simulink model "RM3_rackAndPinion_w_PEC"  (R2024b)
settings: Solver=ode4  StartTime=0  StopTime=200  FixedStep=0.001  MaxStep=0.001  RelTol=1e-3
values from neighbouring files (symbols this model uses):
  simu = simulationClass()    [wecSimInputFile.m]
undefined symbols (not defined in the file or in its folder): body, constraint, diodeA, diodeB1, diodeB2, diodeC, fsw, geometry, heatSinkCth, heatSinkRth, hydroData, igbtA, igbtB1, igbtB2, igbtC, igbtRth, numParallel, pmsg, pto, Vdc, wec, wi
libraries: WECSim_Lib_Body_Elements x2, WECSim_Lib_Frames x1, WECSim_Lib_Constraints x1, WECSim_Lib_PTOs x1
settings Model: Creator=smbar  LastModifiedBy=smbar
settings SolverCC: ZeroCrossControl=DisableAll  AutoInsertRateTranBlk=on
settings DataIOCC: ReturnWorkspaceOutputs=off
settings OptimizationCC: SimCompilerOptimization=on
settings ExplorerConfigSet: SimMechanicsOpenEditorOnUpdate=off

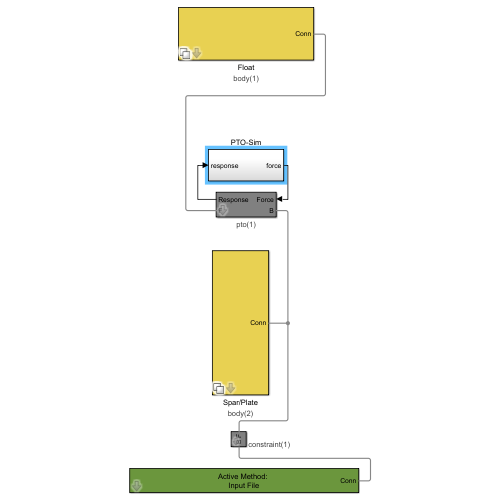
[thumbnail: Simulink's stored preview of the top-level diagram]
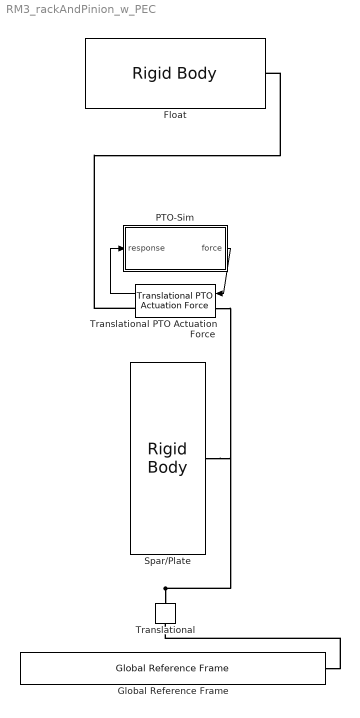
== system RM3_rackAndPinion_w_PEC ==
  Float : WECSim_Lib_Body_Elements/Rigid Body  body=body(1)  h5File=hydroData/*.h5  geometryFile=geometry/*.stl  mass=0  inertia=0 0 0  inertiaProducts=0 0 0  nonHydro=0  nonlinearHydro=0  centerGravity=0 0 0  centerBuoyancy=0 0 0  dof=6  volume=0  QTFs=0  displacement=0 0 0  axis=0 1 0  angle=0  option=0  cd=0 0 0  ca=0 0 0  area=0 0 0  VME=0  rgME=0 0 0  z=0 0 1
  Global Reference Frame : WECSim_Lib_Frames/Global Reference Frame  waves=waves  simu=simu  InputMethod=Input File  InputFile=wecSimInputFile.m  mode=normal  explorer=off  solver=ode4  startTime=0  rampTime=100  endTime=400  dt=0.1  cicEndTime=60  stateSpace=0  WaveClass=regular  height=2.5  period=8  elevationFile=NOT DEFINED  spectrumFile=NOT DEFINED  direction=0  spread=1  spectrumType=NOT DEFINED  phaseSeed=0  option=EqualEnergy
  PTO-Sim : Subsystem
  Spar/Plate : WECSim_Lib_Body_Elements/Rigid Body  body=body(2)  h5File=hydroData/*.h5  geometryFile=geometry/*.stl  mass=0  inertia=0 0 0  inertiaProducts=0 0 0  nonHydro=0  nonlinearHydro=0  centerGravity=0 0 0  centerBuoyancy=0 0 0  dof=6  volume=0  QTFs=0  displacement=0 0 0  axis=0 1 0  angle=0  option=0  cd=0 0 0  ca=0 0 0  area=0 0 0  VME=0  rgME=0 0 0  z=0 0 1
  Translational : WECSim_Lib_Constraints/Translational  constraint=constraint(1)  loc="0  0  0"  displacement=0 0 0  y=0 1 0  z=0 0 1  upperLimitSpecify=off  upperLimitBound=0  upperLimitTransitionRegionWidth=0  upperLimitStiffness=0  upperLimitDamping=0  lowerLimitSpecify=off  lowerLimitBound=0  lowerLimitTransitionRegionWidth=0  lowerLimitStiffness=0  lowerLimitDamping=0
      settings: AttributesFormatString=%<constraint>
  Translational PTO Actuation Force : WECSim_Lib_PTOs/Translational PTO Actuation Force  pto=pto(1)  loc="0  0  0"  stiffness=0  damping=0  equilibriumPosition=0  pretension=0  displacement=0 0 0  y=0 1 0  z=0 0 1  upperLimitSpecify=off  upperLimitBound=0  upperLimitTransitionRegionWidth=0  upperLimitStiffness=0  upperLimitDamping=0  lowerLimitSpecify=off  lowerLimitBound=0  lowerLimitTransitionRegionWidth=0  lowerLimitStiffness=0  lowerLimitDamping=0
      settings: AttributesFormatString=%<pto>
  wires:
  Translational PTO Actuation Force/1 -> PTO-Sim/1(response)
  PTO-Sim/1(force) -> Translational PTO Actuation Force/1
  connections:
  Translational/RConn1 -- Spar/Plate/RConn1 -- Translational PTO Actuation Force/LConn1
  Global Reference Frame/RConn1 -- Translational/LConn1
  Translational PTO Actuation Force/RConn1 -- Float/RConn1

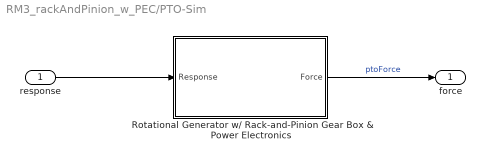
== system RM3_rackAndPinion_w_PEC/PTO-Sim ==
  response : Inport
  Rotational Generator w/ Rack-and-Pinion Gear Box & Power Electronics : Subsystem
  force : Outport  VectorParamsAs1DForOutWhenUnconnected=off
  wires:
  response/1 -> Rotational Generator w/ Rack-and-Pinion Gear Box & Power Electronics/1(Response)
  Rotational Generator w/ Rack-and-Pinion Gear Box & Power Electronics/1(Force) -> force/1  "ptoForce"

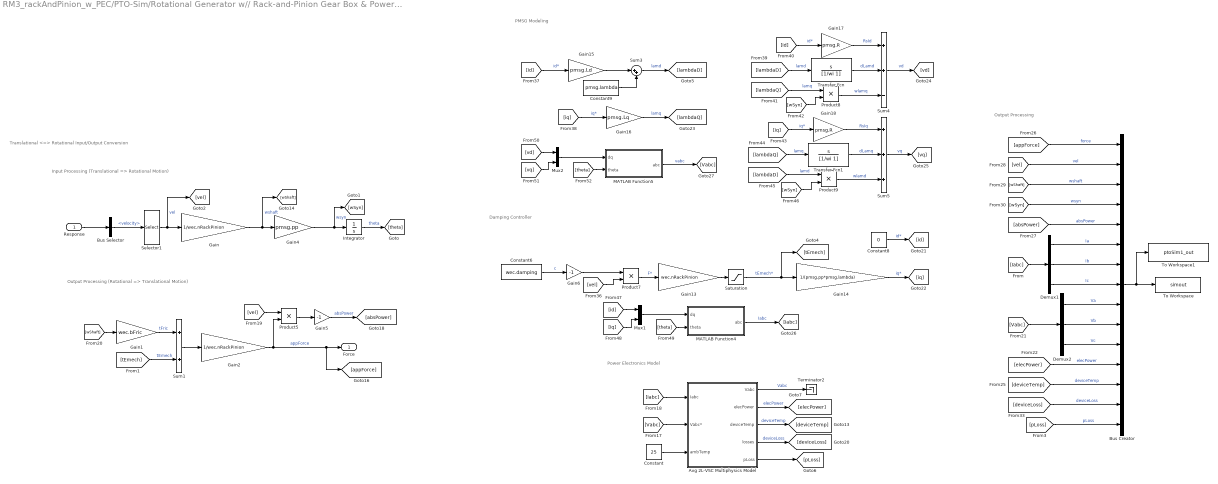
== system RM3_rackAndPinion_w_PEC/PTO-Sim/Rotational Generator w// Rack-and-Pinion Gear Box & Power Electronics ==
  note: Damping Controller
  note: PMSG Modeling
  note: Output Processing
  note: Output Processing (Rotational => Translational Motion)
  note: Input Processing (Translational => Rotational Motion)
  note: Translational <=> Rotational Input/Output Conversion
  note: Power Electronics Model
  Response : Inport
  Avg 2L-VSC Multiphysics Model : Subsystem
  Bus Creator : BusCreator  Inputs=15
  Bus Selector : BusSelector  OutputSignals=velocity
  Constant : Constant  Value=25
  Constant6 : Constant  Value=wec.damping
  Constant8 : Constant  Value=0
  Constant9 : Constant  Value=pmsg.lambda
  Demux1 : Demux  Outputs=3
  Demux2 : Demux  Outputs=3
  Gain : Gain  Gain=1/wec.nRackPinion
  Gain1 : Gain  Gain=wec.bFric
  Gain13 : Gain  Gain=wec.nRackPinion
  Gain14 : Gain  Gain=1/(pmsg.pp*pmsg.lambda)
  Gain15 : Gain  Gain=pmsg.Ld
  Gain16 : Gain  Gain=pmsg.Lq
  Gain17 : Gain  Gain=pmsg.R
  Gain18 : Gain  Gain=pmsg.R
  Gain2 : Gain  Gain=1/wec.nRackPinion
  Gain4 : Gain  Gain=pmsg.pp
  Gain5 : Gain  Gain=-1
  Gain6 : Gain  Gain=-1
  Integrator : Integrator  WrapState=on  WrappedStateUpperValue=2*pi  WrappedStateLowerValue=0
  MATLAB Function4 : MATLAB Function  TreatAsAtomicUnit=on
  MATLAB Function5 : MATLAB Function  TreatAsAtomicUnit=on
  Mux1 : Mux  Inputs=2
  Mux2 : Mux  Inputs=2
  Product{5,7..9} (4 alike) : Product
  Saturation : Saturate  UpperLimit=pmsg.tRated  LowerLimit=-pmsg.tRated
  Selector1 : Selector  InputPortWidth=6  IndexOptions=Index vector (dialog)  Indices=3  OutputSizes=1
  Sum1 : Sum
  Sum3 : Sum  Inputs=|++
  Sum4 : Sum  Inputs=++-
  Sum5 : Sum  Inputs=+++
  Terminator2 : Terminator
  To Workspace : ToWorkspace  VariableName=simout  SaveFormat=Timeseries  SampleTime=-1
  To Workspace1 : ToWorkspace  VariableName=ptoSim1_out  SaveFormat=Structure With Time  SampleTime=simu.dtOut
  Transfer Fcn : TransferFcn  Numerator=[1 0]  Denominator=[1/wi 1]
  Transfer Fcn1 : TransferFcn  Numerator=[1 0]  Denominator=[1/wi 1]
  Force : Outport
  wires:
  Bus Selector/1 -> Selector1/1  "<velocity>"
  Response/1 -> Bus Selector/1
  Selector1/1 -> [vel], Gain/1  "vel"
  Gain4/1 -> Integrator/1, [wSyn]  "wsyn"
  Integrator/1 -> [theta]  "theta"
  [wShaft] -> Gain1/1
  Gain1/1 -> Sum1/1  "tFric"
  Gain2/1 -> [appForce], Force/1, Product5/2  "appForce"
  Sum1/1 -> Gain2/1
  [tEmech] -> Sum1/2  "tEmech"
  [Vabc] -> Avg 2L-VSC Multiphysics Model/2(Vabc*)
  [Iabc] -> Avg 2L-VSC Multiphysics Model/1(Iabc)
  Constant/1 -> Avg 2L-VSC Multiphysics Model/3(ambTemp)
  Avg 2L-VSC Multiphysics Model/1(Vabc) -> Terminator2/1  "Vabc"
  Avg 2L-VSC Multiphysics Model/2(elecPower) -> [elecPower]  "elecPower"
  Avg 2L-VSC Multiphysics Model/3(deviceTemp) -> [deviceTemp]  "deviceTemp"
  Gain/1 -> [wShaft], Gain4/1  "wshaft"
  [vel] -> Product5/1
  Product5/1 -> Gain5/1
  Gain5/1 -> [absPower]  "absPower"
  Bus Creator/1 -> To Workspace1/1, To Workspace/1
  [Iabc] -> Demux1/1
  [Vabc] -> Demux2/1
  Demux2/1 -> Bus Creator/9  "Va"
  [elecPower] -> Bus Creator/12  "elecPower"
  [deviceTemp] -> Bus Creator/13  "deviceTemp"
  Demux2/2 -> Bus Creator/10  "Vb"
  Demux2/3 -> Bus Creator/11  "Vc"
  Demux1/2 -> Bus Creator/7  "Ib"
  Demux1/1 -> Bus Creator/6  "Ia"
  Demux1/3 -> Bus Creator/8  "Ic"
  [appForce] -> Bus Creator/1  "force"
  [vel] -> Bus Creator/2  "vel"
  [wShaft] -> Bus Creator/3  "wshaft"
  [wSyn] -> Bus Creator/4  "wsyn"
  [absPower] -> Bus Creator/5  "absPower"
  [pLoss] -> Bus Creator/15  "pLoss"
  Avg 2L-VSC Multiphysics Model/4(losses) -> [deviceLoss]  "deviceLoss"
  [deviceLoss] -> Bus Creator/14  "deviceLoss"
  [vel] -> Product7/2
  Product7/1 -> Gain13/1  "F*"
  Gain13/1 -> Saturation/1
  Gain14/1 -> [iq]  "iq*"
  [id] -> Gain15/1  "id*"
  Gain15/1 -> Sum3/1
  Constant9/1 -> Sum3/2
  Sum3/1 -> [lambdaD]  "lamd"
  Gain16/1 -> [lambdaQ]  "lamq"
  Constant8/1 -> [id]  "id*"
  [iq] -> Gain16/1  "iq*"
  [lambdaD] -> Transfer Fcn/1  "lamd"
  Transfer Fcn/1 -> Sum4/2  "dLamd"
  [id] -> Gain17/1  "id*"
  [lambdaQ] -> Product8/1  "lamq"
  [wSyn] -> Product8/2
  Gain17/1 -> Sum4/1  "RsId"
  Product8/1 -> Sum4/3  "wlamq"
  Sum4/1 -> [vd]  "vd"
  [iq] -> Gain18/1  "iq*"
  [lambdaQ] -> Transfer Fcn1/1  "lamq"
  Product9/1 -> Sum5/3  "wlamd"
  Transfer Fcn1/1 -> Sum5/2  "dLamq"
  Gain18/1 -> Sum5/1  "RsIq"
  [lambdaD] -> Product9/1  "lamd"
  [wSyn] -> Product9/2
  Sum5/1 -> [vq]  "vq"
  [iq] -> Mux1/2
  [id] -> Mux1/1
  Mux1/1 -> MATLAB Function4/1(dq)
  [theta] -> MATLAB Function4/2(theta)
  MATLAB Function4/1(abc) -> [Iabc]  "Iabc"
  [theta] -> MATLAB Function5/2(theta)
  [vd] -> Mux2/1
  Mux2/1 -> MATLAB Function5/1(dq)
  [vq] -> Mux2/2
  MATLAB Function5/1(abc) -> [Vabc]  "vabc"
  Gain6/1 -> Product7/1
  Constant6/1 -> Gain6/1  "c"
  Saturation/1 -> [tEmech], Gain14/1  "tEmech*"
  Avg 2L-VSC Multiphysics Model/5(pLoss) -> [pLoss]

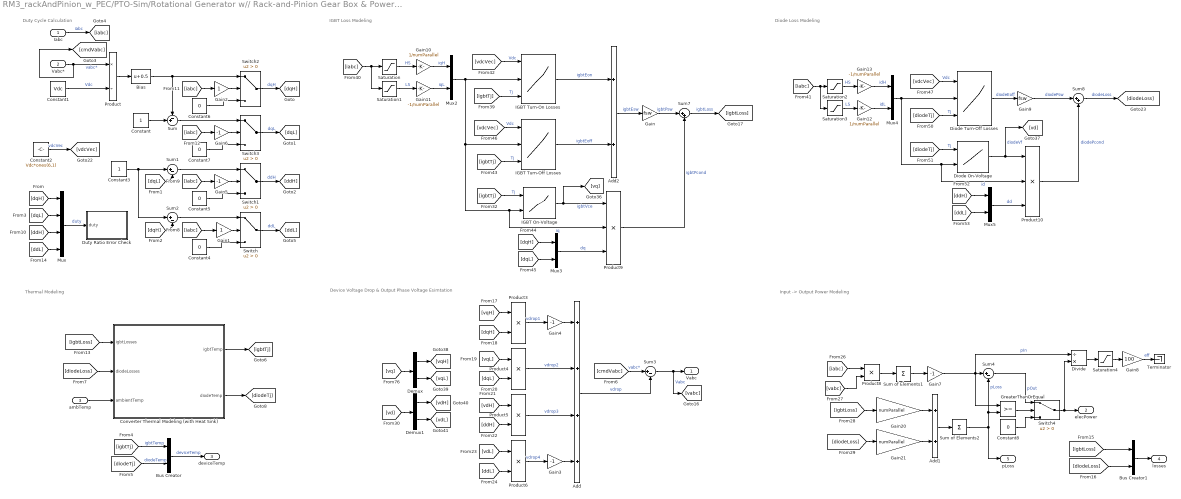
== system RM3_rackAndPinion_w_PEC/PTO-Sim/Rotational Generator w// Rack-and-Pinion Gear Box & Power Electronics/Avg 2L-VSC Multiphysics Model ==
  note: Thermal Modeling
  note: Diode Loss Modeling
  note: IGBT Loss Modeling
  note: Input -> Output Power Modeling
  note: Device Voltage Drop & Output Phase Voltage Esimtation
  note: Duty Cycle Calculation
  Iabc : Inport
  Vabc* : Inport  Port=2
  ambTemp : Inport  Port=3
  Add : Sum  Inputs=++++
  Add1 : Sum
  Add2 : Sum
  Bias : Bias  Bias=0.5  SaturateOnIntegerOverflow=off
  Bus Creator : BusCreator  Inputs=2
  Bus Creator1 : BusCreator  Inputs=2
  Constant : Constant
  Constant1 : Constant  Value=Vdc
  Constant2 : Constant  Value=Vdc*ones(6,1)
  Constant3 : Constant
  Constant{4..8} (5 alike) : Constant  Value=0
  Converter Thermal Modeling (with Heat Sink) : Subsystem
  Demux : Demux  Outputs=2
  Demux1 : Demux  Outputs=2
  Diode On-Voltage : Lookup_n-D  DataSpecification=Lookup table object  LookupTableObject=diodeVonLUT  BreakpointsForDimension3=[5, 7]  Table=reshape(repmat([4 5 6;16 19 20;10 18 23],1,2),[3,3,2])  InternalRulePriority=Speed  RndMeth=Simplest
      settings: InputPortMap=u0,u1
  Diode Turn-Off Losses : Lookup_n-D  NumberOfTableDimensions=3  DataSpecification=Lookup table object  LookupTableObject=diodeEoffLUT  BreakpointsForDimension3=[5, 7]  Table=reshape(repmat([4 5 6;16 19 20;10 18 23],1,2),[3,3,2])  InternalRulePriority=Speed  RndMeth=Simplest
      settings: InputPortMap=u0,u1,u2
  Divide : Product  Inputs=/*
  Duty Ratio Error Check : Subsystem
  Gain : Gain  Gain=fsw
  Gain1 : Gain
  Gain10 : Gain  Gain=1/numParallel
  Gain11 : Gain  Gain=-1/numParallel
  Gain12 : Gain  Gain=1/numParallel
  Gain13 : Gain  Gain=-1/numParallel
  Gain2 : Gain
  Gain20 : Gain  Gain=numParallel
  Gain21 : Gain  Gain=numParallel
  Gain{3..7} (5 alike) : Gain  Gain=-1
  Gain8 : Gain  Gain=100
  Gain9 : Gain  Gain=fsw
  GreaterThanOrEqual : RelationalOperator  OutDataTypeStr=boolean  RndMeth=Simplest  InputSameDT=off
  IGBT On-Voltage : Lookup_n-D  DataSpecification=Lookup table object  LookupTableObject=igbtVonLUT  BreakpointsForDimension3=[5, 7]  Table=reshape(repmat([4 5 6;16 19 20;10 18 23],1,2),[3,3,2])  InternalRulePriority=Speed  RndMeth=Simplest
      settings: InputPortMap=u0,u1
  IGBT Turn-Off Losses : Lookup_n-D  NumberOfTableDimensions=3  DataSpecification=Lookup table object  LookupTableObject=igbtEoffLUT  BreakpointsForDimension3=[5, 7]  Table=reshape(repmat([4 5 6;16 19 20;10 18 23],1,2),[3,3,2])  InternalRulePriority=Speed  RndMeth=Simplest
      settings: InputPortMap=u0,u1,u2
  IGBT Turn-On Losses : Lookup_n-D  NumberOfTableDimensions=3  DataSpecification=Lookup table object  LookupTableObject=igbtEonLUT  BreakpointsForDimension3=[5, 7]  Table=reshape(repmat([4 5 6;16 19 20;10 18 23],1,2),[3,3,2])  InternalRulePriority=Speed  RndMeth=Simplest
      settings: InputPortMap=u0,u1,u2
  Mux : Mux  Inputs=[3 3 3 3]
  Mux{2..5} (4 alike) : Mux  Inputs=2
  Product : Product  Inputs=*/
  Product10 : Product  Inputs=3
  Product{3..6,8} (5 alike) : Product
  Product9 : Product  Inputs=3
  Saturation : Saturate  UpperLimit=inf  LowerLimit=0
  Saturation1 : Saturate  UpperLimit=0  LowerLimit=-inf
  Saturation2 : Saturate  UpperLimit=0  LowerLimit=-inf
  Saturation3 : Saturate  UpperLimit=inf  LowerLimit=0
  Saturation4 : Saturate  UpperLimit=inf  LowerLimit=0
  Sum : Sum  Inputs=-+|
  Sum of Elements1 : Sum  Inputs=+
  Sum of Elements2 : Sum  Inputs=+
  Sum{1..4} (4 alike) : Sum  Inputs=|+-
  Sum7 : Sum  Inputs=|++
  Sum8 : Sum  Inputs=|++
  Switch{,1..4} (5 alike) : Switch  Criteria=u2 > Threshold  SaturateOnIntegerOverflow=off  InputSameDT=off
  Terminator : Terminator
  Vabc : Outport
  elecPower : Outport  Port=2
  deviceTemp : Outport  Port=3
  losses : Outport  Port=4
  pLoss : Outport  Port=5
  wires:
  Iabc/1 -> [iabc]  "iabc"
  Vabc*/1 -> [cmdVabc], Product/1  "vabc*"
  Constant1/1 -> Product/2  "Vdc"
  Sum/1 -> Switch3/1
  Bias/1 -> Sum/1, Switch2/1
  Constant3/1 -> Sum2/1, Sum1/1
  [dqL] -> Sum1/2
  [dqH] -> Sum2/2
  Sum2/1 -> Switch/1
  Constant4/1 -> Switch/3
  Constant5/1 -> Switch1/3
  Switch1/1 -> [ddH]  "ddH"
  [iabc] -> Gain5/1
  Switch/1 -> [ddL]  "ddL"
  Switch2/1 -> [dqH]  "dqH"
  [iabc] -> Gain2/1
  Constant6/1 -> Switch2/3
  Constant7/1 -> Switch3/3
  [iabc] -> Gain6/1
  Switch3/1 -> [dqL]  "dqL"
  Constant/1 -> Sum/2
  Gain2/1 -> Switch2/2
  [iabc] -> Gain1/1
  Gain1/1 -> Switch/2
  [cmdVabc] -> Sum3/1  "vabc*"
  [vqH] -> Product3/1
  [dqH] -> Product3/2
  Product3/1 -> Gain4/1  "vdrop1"
  [vqL] -> Product4/1
  Product4/1 -> Add/2  "vdrop2"
  [dqL] -> Product4/2
  [vdH] -> Product5/1
  Product5/1 -> Add/3  "vdrop3"
  [ddH] -> Product5/2
  [vdL] -> Product6/1
  Product6/1 -> Gain3/1  "vdrop4"
  [ddL] -> Product6/2
  Add/1 -> Sum3/2  "vdrop"
  Gain3/1 -> Add/4
  Gain4/1 -> Add/1
  Sum3/1 -> Vabc/1, [vabc]  "Vabc"
  Sum1/1 -> Switch1/1
  Product8/1 -> Sum of Elements1/1
  [iabc] -> Product8/1
  Sum of Elements1/1 -> Gain7/1
  [diodeLoss] -> Gain21/1
  [igbtLoss] -> Gain20/1
  Add1/1 -> Sum of Elements2/1
  Gain5/1 -> Switch1/2
  Gain6/1 -> Switch3/2
  Sum of Elements2/1 -> Sum4/2, GreaterThanOrEqual/2, pLoss/1  "pLoss"
  [vdcVec] -> IGBT Turn-On Losses/1  "Vdc"
  Mux2/1 -> IGBT Turn-Off Losses/2, Product9/2, IGBT On-Voltage/2, IGBT Turn-On Losses/2  "iq"
  [igbtTj] -> IGBT Turn-On Losses/3  "Tj"
  Mux4/1 -> Product10/2, Diode On-Voltage/2, Diode Turn-Off Losses/2  "id"
  IGBT On-Voltage/1 -> [vq], Product9/1  "igbtVce"
  IGBT Turn-On Losses/1 -> Add2/1  "igbtEon"
  IGBT Turn-Off Losses/1 -> Add2/2  "igbtEoff"
  Diode Turn-Off Losses/1 -> Gain9/1  "diodeEoff"
  Diode On-Voltage/1 -> [vd], Product10/1  "diodeVf"
  Gain11/1 -> Mux2/2  "iqL"
  Constant2/1 -> [vdcVec]  "vdcVec"
  [igbtTj] -> IGBT Turn-Off Losses/3  "Tj"
  [vdcVec] -> IGBT Turn-Off Losses/1  "Vdc"
  [vdcVec] -> Diode Turn-Off Losses/1  "Vdc"
  [diodeTj] -> Diode Turn-Off Losses/3  "Tj"
  [igbtTj] -> IGBT On-Voltage/1  "Tj"
  [dqH] -> Mux3/1
  [dqL] -> Mux3/2
  Mux3/1 -> Product9/3  "dq"
  Add2/1 -> Gain/1  "igbtEsw"
  Gain/1 -> Sum7/1  "igbtPsw"
  Gain9/1 -> Sum8/1  "diodePsw"
  [diodeTj] -> Diode On-Voltage/1  "Tj"
  Mux5/1 -> Product10/3  "dd"
  [ddL] -> Mux5/2
  [ddH] -> Mux5/1
  Saturation/1 -> Gain10/1  "HS"
  Saturation1/1 -> Gain11/1  "LS"
  Gain10/1 -> Mux2/1  "iqH"
  [iabc] -> Saturation1/1, Saturation/1
  Saturation3/1 -> Gain12/1  "LS"
  Gain13/1 -> Mux4/1  "idH"
  Saturation2/1 -> Gain13/1  "HS"
  Gain12/1 -> Mux4/2  "idL"
  [iabc] -> Saturation3/1, Saturation2/1
  Sum7/1 -> [igbtLoss]  "igbtLoss"
  Sum8/1 -> [diodeLoss]  "diodeLoss"
  [vq] -> Demux/1
  Demux/1 -> [vqH]
  Demux/2 -> [vqL]
  [vd] -> Demux1/1
  Demux1/1 -> [vdH]
  Demux1/2 -> [vdL]
  [igbtTj] -> Bus Creator/1  "igbtTemp"
  [diodeTj] -> Bus Creator/2  "diodeTemp"
  Bus Creator/1 -> deviceTemp/1  "deviceTemp"
  Sum4/1 -> Switch4/1  "pOut"
  Gain7/1 -> Divide/1, GreaterThanOrEqual/1, Sum4/1  "pIn"
  Switch4/1 -> elecPower/1, Divide/2
  GreaterThanOrEqual/1 -> Switch4/2
  Constant8/1 -> Switch4/3
  Divide/1 -> Saturation4/1
  Gain8/1 -> Terminator/1  "eff"
  Saturation4/1 -> Gain8/1
  Product10/1 -> Sum8/2  "diodePcond"
  Product9/1 -> Sum7/2  "igbtPcond"
  Gain20/1 -> Add1/1
  Gain21/1 -> Add1/2
  [igbtLoss] -> Converter Thermal Modeling (with Heat Sink)/1(igbtLosses)
  [diodeLoss] -> Converter Thermal Modeling (with Heat Sink)/2(diodeLosses)
  ambTemp/1 -> Converter Thermal Modeling (with Heat Sink)/3(ambientTemp)
  Converter Thermal Modeling (with Heat Sink)/1(igbtTemp) -> [igbtTj]
  Converter Thermal Modeling (with Heat Sink)/2(diodeTemp) -> [diodeTj]
  [dqH] -> Mux/1
  [dqL] -> Mux/2
  [ddH] -> Mux/3
  [ddL] -> Mux/4
  Mux/1 -> Duty Ratio Error Check/1(duty)  "duty"
  Product/1 -> Bias/1
  [diodeLoss] -> Bus Creator1/2
  [igbtLoss] -> Bus Creator1/1
  Bus Creator1/1 -> losses/1
  [vabc] -> Product8/2

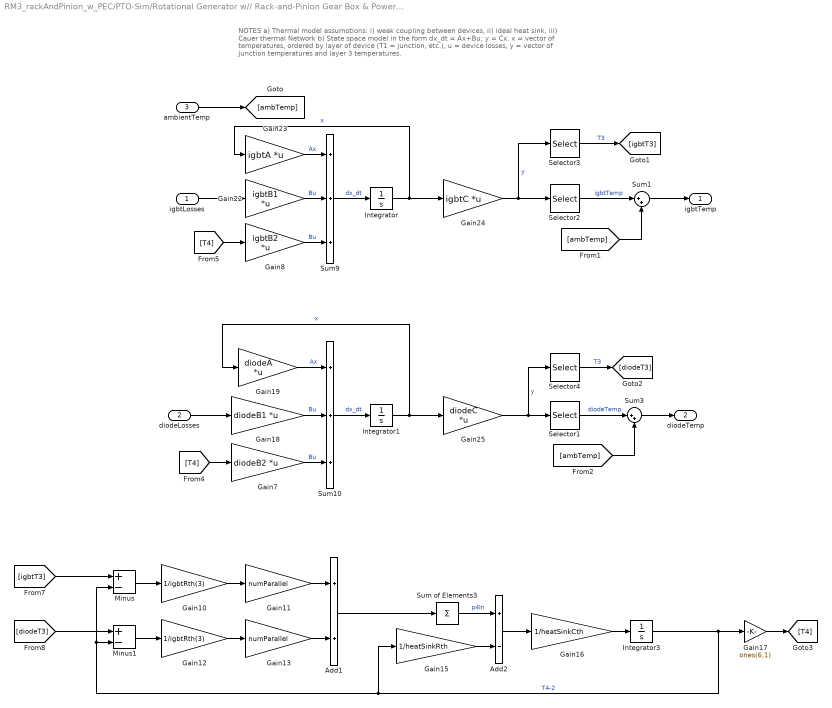
== system RM3_rackAndPinion_w_PEC/PTO-Sim/Rotational Generator w// Rack-and-Pinion Gear Box & Power Electronics/Avg 2L-VSC Multiphysics Model/Converter Thermal Modeling (with Heat Sink) ==
  note: NOTES
      | a) Thermal model assumotions: i) weak coupling between devices, ii) ideal heat sink, iii) Cauer thermal Network
      | b) State space model in the form dx_dt = Ax+Bu; y = Cx. x = vector of temperatures, ordered by layer of device (T1 = junction, etc.), u = device losses, y = vector of junction temperatures and layer 3 temperatures.
  igbtLosses : Inport
  diodeLosses : Inport  Port=2
  ambientTemp : Inport  Port=3
  Add1 : Sum
  Add2 : Sum  Inputs=+-
  Gain10 : Gain  Gain=1/igbtRth(3)
  Gain11 : Gain  Gain=numParallel
  Gain12 : Gain  Gain=1/igbtRth(3)
  Gain13 : Gain  Gain=numParallel
  Gain15 : Gain  Gain=1/heatSinkRth
  Gain16 : Gain  Gain=1/heatSinkCth
  Gain17 : Gain  Gain=ones(6,1)
  Gain18 : Gain  Gain=diodeB1  Multiplication=Matrix(K*u) (u vector)
  Gain19 : Gain  Gain=diodeA  Multiplication=Matrix(K*u) (u vector)
  Gain22 : Gain  Gain=igbtB1  Multiplication=Matrix(K*u) (u vector)
  Gain23 : Gain  Gain=igbtA  Multiplication=Matrix(K*u) (u vector)
  Gain24 : Gain  Gain=igbtC  Multiplication=Matrix(K*u) (u vector)
  Gain25 : Gain  Gain=diodeC  Multiplication=Matrix(K*u) (u vector)
  Gain7 : Gain  Gain=diodeB2  Multiplication=Matrix(K*u) (u vector)
  Gain8 : Gain  Gain=igbtB2  Multiplication=Matrix(K*u) (u vector)
  Integrator : Integrator
  Integrator1 : Integrator
  Integrator3 : Integrator
  Minus : Sum  Inputs=+-
  Minus1 : Sum  Inputs=+-
  Selector1 : Selector  InputPortWidth=18  IndexOptions=Index vector (dialog)  Indices=[1 4 7 10 13 16]  OutputSizes=1
  Selector2 : Selector  InputPortWidth=18  IndexOptions=Index vector (dialog)  Indices=[1 4 7 10 13 16]  OutputSizes=1
  Selector3 : Selector  InputPortWidth=18  IndexOptions=Index vector (dialog)  Indices=[3 6 9 12 15 18]  OutputSizes=1
  Selector4 : Selector  InputPortWidth=18  IndexOptions=Index vector (dialog)  Indices=[3 6 9 12 15 18]  OutputSizes=1
  Sum of Elements3 : Sum  Inputs=+
  Sum1 : Sum  Inputs=|++
  Sum10 : Sum  Inputs=+++
  Sum3 : Sum  Inputs=|++
  Sum9 : Sum  Inputs=+++
  igbtTemp : Outport
  diodeTemp : Outport  Port=2
  wires:
  ambientTemp/1 -> [ambTemp]
  Selector2/1 -> Sum1/1  "igbtTemp"
  Gain18/1 -> Sum10/2  "Bu"
  Selector1/1 -> Sum3/1  "diodeTemp"
  Integrator1/1 -> Gain19/1, Gain25/1  "x"
  Integrator/1 -> Gain23/1, Gain24/1  "x"
  Gain22/1 -> Sum9/2  "Bu"
  Gain23/1 -> Sum9/1  "Ax"
  Sum10/1 -> Integrator1/1  "dx_dt"
  Gain19/1 -> Sum10/1  "Ax"
  Sum9/1 -> Integrator/1  "dx_dt"
  Selector3/1 -> [igbtT3]  "T3"
  Selector4/1 -> [diodeT3]  "T3"
  [T4] -> Gain7/1
  Gain7/1 -> Sum10/3  "Bu"
  [T4] -> Gain8/1
  Gain8/1 -> Sum9/3  "Bu"
  igbtLosses/1 -> Gain22/1
  diodeLosses/1 -> Gain18/1
  [igbtT3] -> Minus/1
  Minus/1 -> Gain10/1
  Gain10/1 -> Gain11/1
  Gain11/1 -> Add1/1
  [diodeT3] -> Minus1/1
  Gain12/1 -> Gain13/1
  Minus1/1 -> Gain12/1
  Gain13/1 -> Add1/2
  Add1/1 -> Sum of Elements3/1
  Sum of Elements3/1 -> Add2/1  "p4In"
  Gain15/1 -> Add2/2
  Add2/1 -> Gain16/1
  Gain16/1 -> Integrator3/1
  Gain17/1 -> [T4]
  Integrator3/1 -> Minus1/2, Minus/2, Gain15/1, Gain17/1  "T4-2"
  Gain25/1 -> Selector4/1, Selector1/1  "y"
  Gain24/1 -> Selector2/1, Selector3/1  "y"
  [ambTemp] -> Sum1/2
  Sum1/1 -> igbtTemp/1
  Sum3/1 -> diodeTemp/1
  [ambTemp] -> Sum3/2

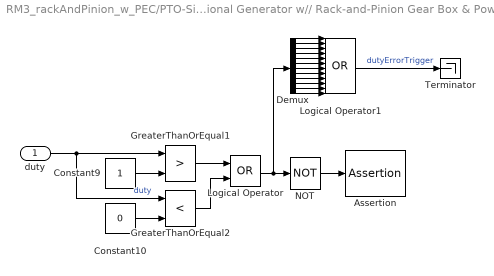
== system RM3_rackAndPinion_w_PEC/PTO-Sim/Rotational Generator w// Rack-and-Pinion Gear Box & Power Electronics/Avg 2L-VSC Multiphysics Model/Duty Ratio Error Check ==
  duty : Inport
  Assertion : Assertion
  Constant10 : Constant  Value=0
  Constant9 : Constant
  Demux : Demux  Outputs=12
  GreaterThanOrEqual1 : RelationalOperator  Operator=>  OutDataTypeStr=boolean  RndMeth=Simplest  InputSameDT=off
  GreaterThanOrEqual2 : RelationalOperator  Operator=<  OutDataTypeStr=boolean  RndMeth=Simplest  InputSameDT=off
  Logical Operator : Logic  Operator=OR  AllPortsSameDT=off  OutDataTypeStr=boolean
  Logical Operator1 : Logic  Operator=OR  Inputs=12  AllPortsSameDT=off  OutDataTypeStr=boolean
  NOT : Logic  Operator=NOT  IconShape=distinctive  AllPortsSameDT=off  OutDataTypeStr=boolean
  Terminator : Terminator
  wires:
  Constant9/1 -> GreaterThanOrEqual1/2
  Constant10/1 -> GreaterThanOrEqual2/2
  GreaterThanOrEqual2/1 -> Logical Operator/2
  Logical Operator/1 -> Demux/1, NOT/1
  duty/1 -> GreaterThanOrEqual2/1, GreaterThanOrEqual1/1  "duty"
  GreaterThanOrEqual1/1 -> Logical Operator/1
  NOT/1 -> Assertion/1
  Logical Operator1/1 -> Terminator/1  "dutyErrorTrigger"
  Demux/1 -> Logical Operator1/1
  Demux/2 -> Logical Operator1/2
  Demux/3 -> Logical Operator1/3
  Demux/4 -> Logical Operator1/4
  Demux/5 -> Logical Operator1/5
  Demux/6 -> Logical Operator1/6
  Demux/7 -> Logical Operator1/7
  Demux/8 -> Logical Operator1/8
  Demux/9 -> Logical Operator1/9
  Demux/10 -> Logical Operator1/10
  Demux/11 -> Logical Operator1/11
  Demux/12 -> Logical Operator1/12

== matlab function RM3_rackAndPinion_w_PEC/PTO-Sim/Rotational Generator w// Rack-and-Pinion Gear Box & Power Electronics/MATLAB Function5 ==
  data: dq input; abc output; theta input
function abc  = dq_to_abc(dq, theta)
% DQ_TO_ABC Power Invariant Inverse dq Transform
% Takes dq input along with current electrical angle, and converts to the
% equivalent abc value. 

abc = zeros(3,1);

abc(1) = sqrt(2/3) * (cos(theta)*dq(1) - sin(theta)*dq(2));
abc(2) = sqrt(2/3) * (cos(theta-2*pi/3)*dq(1) - sin(theta-2*pi/3)*dq(2));
abc(3) = sqrt(2/3) * (cos(theta-4*pi/3)*dq(1) - sin(theta-4*pi/3)*dq(2));

end

== matlab function RM3_rackAndPinion_w_PEC/PTO-Sim/Rotational Generator w// Rack-and-Pinion Gear Box & Power Electronics/MATLAB Function4 ==
  data: dq input; abc output; theta input
function abc  = dq_to_abc(dq, theta)
% DQ_TO_ABC Power Invariant Inverse dq Transform
% Takes dq input along with current electrical angle, and converts to the
% equivalent abc value. 

abc = zeros(3,1);

abc(1) = sqrt(2/3) * (cos(theta)*dq(1) - sin(theta)*dq(2));
abc(2) = sqrt(2/3) * (cos(theta-2*pi/3)*dq(1) - sin(theta-2*pi/3)*dq(2));
abc(3) = sqrt(2/3) * (cos(theta-4*pi/3)*dq(1) - sin(theta-4*pi/3)*dq(2));

end
